simulink model "UPS_Harness"  (R2025b)
settings: Solver=VariableStepAuto  StartTime=0.0  StopTime=10.0  RelTol=1e-3
PreLoadFcn:
  | UPSHarnessParam
undefined symbols (not defined in the file): ctLimitDelayTime, DiscIntNeverNeededParam, ee_sli_rtmsupport, gcbh, powerTau, Ts, ups
libraries: eeGeneralControl x18, nesl_utility x17, simulink x17, fl_lib x15, ee_lib x13, eeTransforms x7, nesl_utility_internal x4, slpidlib x3, eeSinusoidalMeasurementV2 x3, simulink_extras x3, batteryecm_lib x1
(part 1 of 3)
settings Model: SimulationMode=accelerator  Creator=skota  LastModifiedBy=skota
settings SimscapeCC: SimscapeNominalValues="[{\"value\":\"1\",\"unit\":\"A\"},{\"value\":\"1\",\"unit\":\"bar\"},{\"value\":\"1\",\"unit\":\"cm^2\"},{\"value\":\"1\",\"unit\":\"cm^3/s\"},{\"value\":\"1\",\"unit\":\"kJ/kg\"},{\"value\":\"1\",\"unit\":\"kW\"},{\"value\":\"1\",\"unit\":\"l\"},{\"value\":\"1\",\"unit\":\"N\"},{\"value\":\"1\",\"unit\":\"N*m\"},{\"value\":\"1\",\"unit\":\"V\"},{\"value\":\"0.001\",\"unit\":\"Wb\"}]"  SimscapeLogType=all  SimscapeLogDataHistory=10000.0

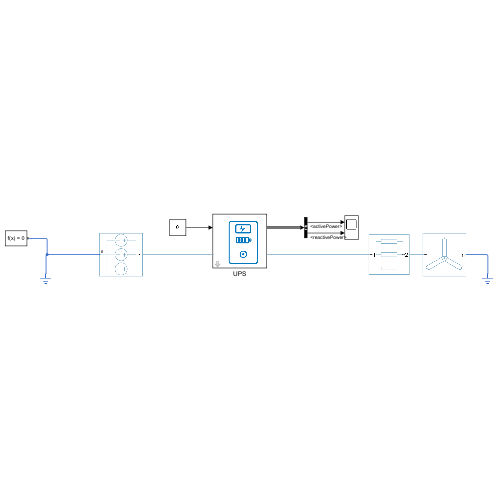
[thumbnail: Simulink's stored preview of the top-level diagram]
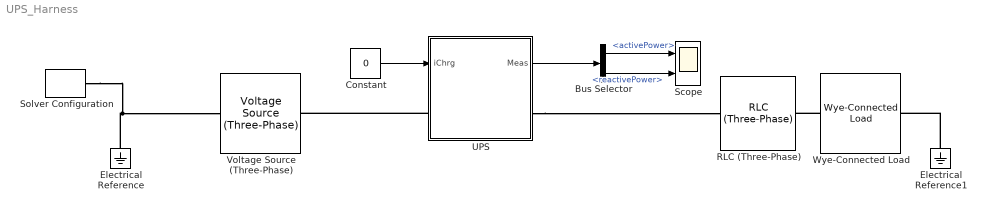
== system UPS_Harness ==
  Bus Selector : BusSelector  OutputSignals=activePower,reactivePower
  Constant : Constant  Value=0
  Electrical Reference : fl_lib/Electrical/Electrical Elements/Electrical Reference
  Electrical Reference1 : fl_lib/Electrical/Electrical Elements/Electrical Reference
  RLC (Three-Phase) : ee_lib/Passive/RLC Assemblies/RLC (Three-Phase)  port_option=ee.enum.threePhasePort.composite  component_structure=ee.enum.rlc.structure.SeriesRL  R=1e-3%1e-4 Ohm  L=1e-6%1e-6 H  C=1e-6 F  R_parasitic=0 Ohm  G_parasitic=0 1/Ohm  IL_specify=on  IL_priority=None  IL=[0, 0, 0] A  IL_nominal_specify=off  IL_nominal_value=1  IL_nominal_unit=A  VC_specify=off  VC_priority=High  VC=[0, 0, 0] V  VC_nominal_specify=off  VC_nominal_value=1  VC_nominal_unit=V
      settings: InternalSimscapePortConfiguration="{\"Bottom\":[],\"Left\":[{\"id\":\"N1\",\"label\":\"~1\",\"type\":\"foundation.electrical.three_phase\"}],\"Right\":[{\"id\":\"N2\",\"label\":\"~2\",\"type\":\"foundation.electrical.three_phase\"}],\"Top\":[]}"
  Scope : Scope  NumInputPorts=2
      settings: ActiveDisplayYMinimum=-0.21717688622608089  ActiveDisplayYMaximum=1.9545919760347286
  Solver Configuration : nesl_utility/Solver Configuration  PhysicalDomain=network_engine_domain  SubClassName=solver  LeftPortType=input  RightPortType=generic  Tones=[]  Harmonics=[]  SimulateNoise=off  Profile=off  UseLocalSampling=off  EnableSwitchedLinearOptims=on  FrequencyDomain=off  UseCCode=off  RelTol=0.001  AbsTol=0.001  MinStep=1e-09  ToWorkspace=off  RevertToSquareIcSolve=off  NumHomotopyIterations=100  PhasorMode=off  PhasorModeNumHarmonics=1  ConsistencySolver=NEWTON_XTOL_AFTER_FTOL  IndexReductionMethod=None  DoDC=off  ResidualTolerance=1e-09  ConsistencyTolSource=GLOBAL  ConsistencyAbsTol=0.001  ConsistencyRelTol=0.001  ConsistencyTolFactor=1e3  UseLocalSolver=on  LocalSolverChoice=NE_BACKWARD_EULER_ADVANCER  ResolveIndetEquations=off  FunctionEvalNumThread=1  LocalSolverSampleTime=5e-05  DoFixedCost=on  MaxNonlinIter=1  MaxModeIter=2  ComputeImpulses=off  ImpulseIterations=2  LinearAlgebra=auto  LinearAlgebraNumThread=0  EquationFormulation=NE_TIME_EF  DelaysMemoryBudget=1024  AutomaticFiltering=off  FilteringTimeConstant=0.001  PartitionStorageMethod=AS_NEEDED  PartitionMemoryBudget=1024  PartitionMethod=ROBUST  MultibodyUseLocalSolver=off  MultibodyLocalSolverChoice=ODE1  MultibodyLocalSolverSampleTime=0.001
  UPS : Subsystem  VariantControl=Detailed  mask(Double-conversion Uniterrupted Power Supply (UPS)){plantRating=ups.rating, Vac=ups.Vac, frequency=ups.frequency, baseVoltageDC=ups.Vdc, sampleTime=ups.sampleTime, filterInductanceAFE=ups.AFE.filterInductance, filterResistanceAFE=ups.AFE.filterResistance/10, capacitance=ups.DCBus.capacitance, vBattNom=ups.batt.Vnom, iBatt=ups.batt.iRated, vBattMax=ups.batt.VMax, droopGain=ups.DCBus.droop, rampRate=ups.batt.rampRate, vGridMin=ups.DCBus.gridThreshold, vDCThreshold=ups.DCBus.VThreshold, initialMode=ups.batt.initialMode, kpDC=500%ups.DCBus.kpConverter/10, kiDC=500%ups.DCBus.kiConverter/10, bessConverterEfficiency=ups.DCBus.converterEff, filterInductance=ups.inverter.filterInductance, filterResistance=ups.inverter.filterResistance}
      mask prompts: plantRating "UPS Rating (kW)"; Vac "Rated AC side voltage (phase-phase RMS) (V)"; frequency "Rated electrical frequency at AC side (Hz)"; baseVoltageDC "Voltage on DC side (V)"; sampleTime "Sample time (s)"; filterInductanceAFE "Filter inductance (H)"; filterResistanceAFE "Filter resistance (Ohm)"; capacitance "Capacitance (F)"; vBattNom "Battery nominal voltage (V)"; iBatt "Battery rated current (A)"; vBattMax "Maximum battery voltage (V)"; droopGain "DC bus droop gain"; rampRate "Ramp rate for battery discharge"; vGridMin "Minimum grid voltage (V)"; vDCThreshold "Threshold DC Bus voltage (V)"; initialMode "Initial operating mode"; kpDC "DC-DC Converter proportional gain"; kiDC "DC-DC Converter integral gain"; bessConverterEfficiency "DC-DC converter efficiency (%)"; filterInductance "Filter inductance (H)"; filterResistance "Filter series resistance (Ohm)"
      mask help: This block models a double conversion uninterruptible power supply that continuously supplies the load through an inverter. It isolates the load from input disturbances and uses a battery on the DC link to maintain uninterrupted power during input outages.
      mask Help: web('UPS.html')
      mask DialogControl generalDetailed Prompt: General
      mask DialogControl Container9 Prompt: Active Front End
      mask DialogControl editRectifier Prompt: Edit converter parameters
      mask DialogControl editRectifier Callback:
      | blockPath = [gcb,'/','Rectifier','/','AC-DC Converter'];
      |     component.mask.openBlock(blockPath);
      mask DialogControl configureAFEController Prompt: Edit AFE controller
      mask DialogControl configureAFEController Callback:
      | blockPath = [gcb,'/','Rectifier','/','PFC Rectifier Controller'];
      |     component.mask.openBlock(blockPath);
      mask DialogControl cellDetailed Prompt: DC Link
      mask DialogControl configureBattery Prompt: Edit battery parameters
      mask DialogControl configureBattery Callback:
      | blockPath = [gcb,'/','DC-Link','/','BESS','/','Battery'] ;
      |     component.mask.openBlock(blockPath);
      mask DialogControl controllerDetailed Prompt: Inverter
      mask DialogControl editInverter Prompt: Edit converter parameters
      mask DialogControl editInverter Callback:
      | blockPath = [gcb,'/','Inverter','/','DC- AC Converter'];
      |     component.mask.openBlock(blockPath);
      mask DialogControl editInverterController Prompt: Edit inverter controller
      mask DialogControl editInverterController Callback:
      | blockPath = [gcb,'/','Inverter','/','Inverter Controller'] ;
      |     component.mask.openBlock(blockPath);
  Voltage Source (Three-Phase) : ee_lib/Sources/Voltage Source (Three-Phase)  vline_rms=480 V  shift=0 deg  freq=60 Hz  impedance_option=1  SShortCircuit=100e6 A*V  XR=15  R=0.01 Ohm  L=3.97e-4 H  harmonic_option=0  harmonic_orders=[5, 7, 11, 13]  harmonic_ratios=[.1, .1, .1, .1]  G_parasitic=0 1/Ohm  I_specify=off  I_priority=None  I=[0, 0, 0] A  I_nominal_specify=off  I_nominal_value=1  I_nominal_unit=A
  Wye-Connected Load : ee_lib/Passive/RLC Assemblies/Wye-Connected Load  port_option=ee.enum.threePhasePort.composite  parameterization=ee.enum.rlc.parameterization.ratedpower  component_structure=ee.enum.rlc.structure.R  component_structure_PQ=ee.enum.rlc.structure.R  R=1 Ohm  L=1e-3 H  C=1e-6 F  VRated=480 V  FRated=60 Hz  P=5e6 W  Qpos=1e2 A*V  Qneg=-1e2 A*V  R_parasitic=0 Ohm  G_parasitic=0 1/Ohm  R_parasitic_PQ=0 Ohm  G_parasitic_PQ=0 1/Ohm  Vmag0=24e3 V  Vang0=0 deg  Freq0=60 Hz  IL_specify=off  IL_priority=High  IL=[0, 0, 0] A  IL_nominal_specify=off  IL_nominal_value=1  IL_nominal_unit=A  VC_specify=off  VC_priority=High  VC=[0, 0, 0] V  VC_nominal_specify=off  VC_nominal_value=1  VC_nominal_unit=V
  wires:
  Constant/1 -> UPS/1(iChrg)
  UPS/1(Meas) -> Bus Selector/1
  Bus Selector/1 -> Scope/1  "<activePower>"
  Bus Selector/2 -> Scope/2  "<reactivePower>"
  connections:
  UPS/LConn1 -- Voltage Source (Three-Phase)/RConn1
  Electrical Reference/LConn1 -- Solver Configuration/RConn1 -- Voltage Source (Three-Phase)/LConn1
  UPS/RConn1 -- RLC (Three-Phase)/LConn1
  Wye-Connected Load/LConn1 -- RLC (Three-Phase)/RConn1
  Electrical Reference1/LConn1 -- Wye-Connected Load/RConn1

== system UPS_Harness/UPS ==
  iChrg : Inport
  DC-Link : Subsystem
      settings: CopyFcn=set_param(gcbh,'LinkStatus','none');
      mask Display: image('DCBusbattery_1_1.png');
  Inverter : Subsystem
      settings: PortSchema="{\"entries\":[{\"content\":{\"sides\":[{\"content\":{\"connectorIds\":[\"LConn1\",\"Out1\"]},\"type\":\"ConnectorPlacement.EquallySpacedRectSide\",\"uuid\":\"30eca24e-4a0d-4322-ab8d-7623f6b77d91\"},{\"content\":{\"connectorIds\":[\"In1\",\"RConn1\",\"RConn2\"],\"side\":\"RIGHT\"},\"type\":\"ConnectorPlacement.EquallySpacedRectSide\",\"uuid\":\"08a32252-dd7d-4c32-87e9-6b7a03d2f0b7\"},{\"content\":{\"side\":\"TOP\"},\"type\":\"ConnectorPlacement.EquallySpacedRectSide\",\"uuid\":\"b32a0ebb-b906-46f8-8fa8-e8ceac70a0fa\"}]},\"type\":\"ConnectorPlacement.EquallySpacedConnector\",\"uuid\":\"2dde14a6-acee-4d4e-9286-e85271f40ce0\"}],\"packageUris\":[\"http://schema.mathworks.com/mf0/Connector/R2020b\"],\"version\":\"1.0\"}"
      mask Display: image('Copy_2_of_Inverter.png');
  Rectifier : Subsystem
      mask Display: image('rectifier_1_1.png');
  ABC : PMIOPort  Side=Left
  ~ : PMIOPort  Port=2  Side=Right
  Meas : Outport
  wires:
  DC-Link/1(Meas) -> Rectifier/1(Meas), Inverter/1(DCMeas)
  Rectifier/1(Id) -> DC-Link/2(iPFC)
  iChrg/1 -> DC-Link/1(iChrg)
  Inverter/1(Meas) -> Meas/1
  Rectifier/2(V) -> DC-Link/3(vPCC)
  Rectifier/3(Brk) -> DC-Link/4(Brk)
  connections:
  Rectifier/RConn1 -- DC-Link/LConn1
  Rectifier/RConn2 -- DC-Link/LConn2
  Rectifier/LConn1 -- ABC/RConn1
  Inverter/LConn1 -- ~/RConn1
  DC-Link/RConn1 -- Inverter/RConn1
  Inverter/RConn2 -- DC-Link/RConn2

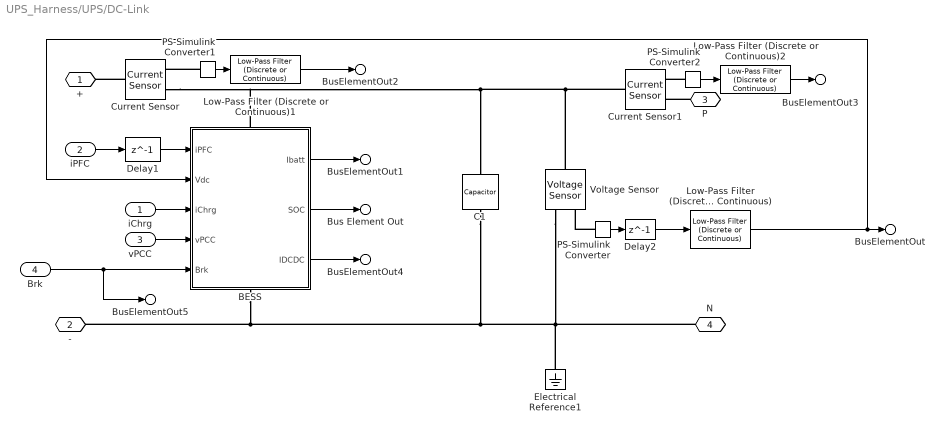
== system UPS_Harness/UPS/DC-Link ==
  iChrg : Inport
  iPFC : Inport  Port=2
  vPCC : Inport  Port=3
  Brk : Inport  Port=4
  BESS : Subsystem
      settings: PortSchema="{\"entries\":[{\"content\":{\"sides\":[{\"content\":{\"connectorIds\":[\"LConn1\"]},\"type\":\"ConnectorPlacement.EquallySpacedRectSide\",\"uuid\":\"dc16109c-3681-46df-aa2d-40033a424f4f\"},{\"content\":{\"connectorIds\":[\"RConn1\"],\"side\":\"RIGHT\"},\"type\":\"ConnectorPlacement.EquallySpacedRectSide\",\"uuid\":\"5490aea4-59f2-45ea-9bac-3971cd260353\"},{\"content\":{\"connectorIds\":[\"Out1\",\"Out2\",\"Out3\"],\"side\":\"TOP\"},\"type\":\"ConnectorPlacement.EquallySpacedRectSide\",\"uuid\":\"92b5185c-680a-4a4f-a590-9680bdd408ad\"},{\"content\":{\"connectorIds\":[\"In1\",\"In2\",\"In3\",\"In4\",\"In5\"],\"side\":\"BOTTOM\"},\"type\":\"ConnectorPlacement.EquallySpacedRectSide\",\"uuid\":\"bb2f2b82-1e61-49ed-8567-aad9343e236f\"}]},\"type\":\"ConnectorPlacement.EquallySpacedConnector\",\"uuid\":\"c23d7033-d24f-41ec-a8dd-f02fcfba4177\"}],\"packageUris\":[\"http://schema.mathworks.com/mf0/Connector/R2020b\"],\"version\":\"1.0\"}"
  C1 : fl_lib/Electrical/Electrical Elements/Capacitor  c=capacitance F  r=1e-3 Ohm  g=0 1/Ohm  i_specify=on  i_priority=None  i=0 A  i_nominal_specify=off  i_nominal_value=1  i_nominal_unit=A  v_specify=off  v_priority=High  v=0 V  v_nominal_specify=off  v_nominal_value=1  v_nominal_unit=V  vc_specify=on  vc_priority=None  vc=baseVoltageDC V  vc_nominal_specify=off  vc_nominal_value=1  vc_nominal_unit=V
  Current Sensor : fl_lib/Electrical/Electrical Sensors/Current Sensor
  Current Sensor1 : fl_lib/Electrical/Electrical Sensors/Current Sensor
  Delay1 : Delay  DelayLength=1  InitialCondition=0.5
  Delay2 : Delay  DelayLength=1  InitialCondition=baseVoltageDC
  Electrical Reference1 : fl_lib/Electrical/Electrical Elements/Electrical Reference
  Low-Pass Filter (Discrete or Continuous) : eeGeneralControl/Low-Pass Filter (Discrete or Continuous)  K=1  T=0.001  B=inf  A=-inf  init_option=Inherited from block input  x0=0  Ts=-1
  Low-Pass Filter (Discrete or Continuous)1 : eeGeneralControl/Low-Pass Filter (Discrete or Continuous)  K=1  T=0.001  B=inf  A=-inf  init_option=Inherited from block input  x0=0  Ts=-1
  Low-Pass Filter (Discrete or Continuous)2 : eeGeneralControl/Low-Pass Filter (Discrete or Continuous)  K=1  T=0.001  B=inf  A=-inf  init_option=Inherited from block input  x0=0  Ts=-1
  PS-Simulink Converter : nesl_utility/PS-Simulink Converter  PhysicalDomain=network_engine_domain  SubClassName=ps_output  LeftPortType=input  RightPortType=output  PseudoPeriodic=off  Frequencies=[]  VectorFormat=inherit  Unit=inherit  AffineConversion=off
  PS-Simulink Converter1 : nesl_utility/PS-Simulink Converter  PhysicalDomain=network_engine_domain  SubClassName=ps_output  LeftPortType=input  RightPortType=output  PseudoPeriodic=off  Frequencies=[]  VectorFormat=inherit  Unit=inherit  AffineConversion=off
  PS-Simulink Converter2 : nesl_utility/PS-Simulink Converter  PhysicalDomain=network_engine_domain  SubClassName=ps_output  LeftPortType=input  RightPortType=output  PseudoPeriodic=off  Frequencies=[]  VectorFormat=inherit  Unit=inherit  AffineConversion=off
  Voltage Sensor : fl_lib/Electrical/Electrical Sensors/Voltage Sensor
  + : PMIOPort  Side=Left
  - : PMIOPort  Port=2  Side=Left
  P : PMIOPort  Port=3  Side=Right
  N : PMIOPort  Port=4  Side=Right
  Bus Element Out : Outport  PortName=Meas  Element=SOC
  BusElementOut : Outport  PortName=Meas  Element=Vdc
  BusElementOut1 : Outport  PortName=Meas  Element=Ibatt
  BusElementOut2 : Outport  PortName=Meas  Element=Idc
  BusElementOut3 : Outport  PortName=Meas  Element=ILoad
  BusElementOut4 : Outport  PortName=Meas  Element=IDCDC
  BusElementOut5 : Outport  PortName=Meas  Element=UPSBrK
  wires:
  iPFC/1 -> Delay1/1
  Delay2/1 -> Low-Pass Filter (Discrete or Continuous)/1
  iChrg/1 -> BESS/3(iChrg)
  Delay1/1 -> BESS/1(iPFC)
  PS-Simulink Converter/1 -> Delay2/1
  BESS/1(Ibatt) -> BusElementOut1/1
  vPCC/1 -> BESS/4(vPCC)
  Brk/1 -> BusElementOut5/1, BESS/5(Brk)
  BESS/2(SOC) -> Bus Element Out/1
  Low-Pass Filter (Discrete or Continuous)/1 -> BESS/2(Vdc), BusElementOut/1
  PS-Simulink Converter1/1 -> Low-Pass Filter (Discrete or Continuous)1/1
  PS-Simulink Converter2/1 -> Low-Pass Filter (Discrete or Continuous)2/1
  Low-Pass Filter (Discrete or Continuous)2/1 -> BusElementOut3/1
  Low-Pass Filter (Discrete or Continuous)1/1 -> BusElementOut2/1
  BESS/3(IDCDC) -> BusElementOut4/1
  connections:
  Electrical Reference1/LConn1 -- N/RConn1 -- Voltage Sensor/RConn2 -- C1/RConn1 -- BESS/RConn1 -- -/RConn1
  PS-Simulink Converter/LConn1 -- Voltage Sensor/RConn1
  Voltage Sensor/LConn1 -- Current Sensor1/LConn1 -- C1/LConn1 -- Current Sensor/RConn2 -- BESS/LConn1
  PS-Simulink Converter1/LConn1 -- Current Sensor/RConn1
  P/RConn1 -- Current Sensor1/RConn2
  PS-Simulink Converter2/LConn1 -- Current Sensor1/RConn1
  Current Sensor/LConn1 -- +/RConn1

== system UPS_Harness/UPS/Inverter ==
  DCMeas : Inport
  DC- AC Converter : ee_lib/Semiconductors & Converters/Converters/Average-Value Voltage Source Converter (Three-Phase)  port_option=ee.enum.threePhasePort.composite  frequency_option=ee.enum.converters.frequency.variable  input_option=ee.enum.converters.inputOption.ModWave  FRated=60 Hz  losses_parameterization=ee.enum.converters.losses.fixed  Pfixed=0.5 W  ks=0.01  kc1=1.7 V  kc2=0.01 Ohm  Ploss_vect=[100, 800, 1870, 3250, 4900] W  Irms_vect=[10, 100, 200, 300, 400] A  Vdc_nom=300 V  thermal_mass=30000 J/K  temperature_specify=off  temperature_priority=High  temperature=298.15 K  temperature_nominal_specify=off  temperature_nominal_value=1  temperature_nominal_unit=K
      settings: InternalSimscapePortConfiguration="{\"Bottom\":[],\"Left\":[{\"id\":\"ModWave\",\"label\":\"ModWave\",\"type\":\"input\"},{\"id\":\"N\",\"label\":\"~\",\"type\":\"foundation.electrical.three_phase\"}],\"Right\":[{\"id\":\"p\",\"label\":\"+\",\"type\":\"foundation.electrical.electrical\"},{\"id\":\"n\",\"label\":\"-\",\"type\":\"foundation.electrical.electrical\"}],\"Top\":[]}"
  Filter & Measurements : Subsystem
      settings: PortSchema="{\"entries\":[{\"content\":{\"sides\":[{\"content\":{\"connectorIds\":[\"LConn1\",\"In1\"]},\"type\":\"ConnectorPlacement.EquallySpacedRectSide\",\"uuid\":\"460c57c7-bd36-455c-a026-acc96216539a\"},{\"content\":{\"connectorIds\":[\"Out1\",\"Out2\",\"RConn1\"],\"side\":\"RIGHT\"},\"type\":\"ConnectorPlacement.EquallySpacedRectSide\",\"uuid\":\"ae96aff3-eaea-4e67-97f2-c12a1605f490\"},{\"content\":{\"side\":\"TOP\"},\"type\":\"ConnectorPlacement.EquallySpacedRectSide\",\"uuid\":\"723b0a2f-7df5-41f2-b267-8daf9f0832d8\"}]},\"type\":\"ConnectorPlacement.EquallySpacedConnector\",\"uuid\":\"b3aac9a5-3f98-4392-99ca-65ef3ff3ee74\"}],\"packageUris\":[\"http://schema.mathworks.com/mf0/Connector/R2020b\"],\"version\":\"1.0\"}"
  Inverter Controller : Subsystem  VariantControl=Grid Forming  mask(UPS Controller){measSampleTime=ups.sampleTime, dcBusVoltage=baseVoltageDC, powerFreq=frequency, girdLineVoltage=Vac, power=plantRating*1000, fDroop=ups.inverter.fDroop, vDroop=ups.inverter.vDroop, vdPGain=ups.inverter.kpVd, VdIGain=ups.inverter.kiVd, VdMaxCt=ups.inverter.IMaxVd, VqPGain=ups.inverter.kpVq, VqIGain=ups.inverter.kiVq, VqMaxCt=ups.inverter.IMaxVd, VdMinCt=ups.inverter.IMinVd, VqMinCt=ups.inverter.IMinVd, vdvqLPFTimeConst=ups.sampleTime*100, voltControlTs=ups.sampleTime, currentControlTs=ups.sampleTime, IdPGain=ups.inverter.kpId, IdIGain=ups.inverter.kiId, IqPGain=ups.inverter.kpIq, IqIGain=ups.inverter.kiIq, filterInductance=filterInductance, currentLimitMethod=Virtual impedance, maxSatCurrentLimit=ups.iLimit.value, ctLimitXbyR=ups.iLimit.XByR, ctLimitVirtualImp=ups.iLimit.resistance}
      mask prompts: measSampleTime "Measurement sample time"; dcBusVoltage "DC bus voltage"; powerFreq "Grid frequency (Hz)"; girdLineVoltage "Grid line voltage (V)"; power "Converter power (VA)"; fDroop "Frequency droop"; vDroop "Voltage droop"; vdPGain "Vd proportional gain"; VdIGain "Vd integral gain"; VdMaxCt "Vd maximum current limit (A)"; VqPGain "Vq proportional gain"; VqIGain "Vq integral gain"; VqMaxCt "Vq maximum current limit (A)"; VdMinCt "Vd minimum current limit  (A)"; VqMinCt "Vq minimum current limit  (A)"; vdvqLPFTimeConst "Voltage measurement filter time constant (s)"; voltControlTs "Controller sample time (s)"; currentControlTs "Controller sample time (s)"; IdPGain "Id proportional gain"; IdIGain "Id integral gain"; IqPGain "Iq proportional gain"; IqIGain "Iq integral gain"; filterInductance "Filter inductance (H)"; currentLimitMethod "Current limiting method"; maxSatCurrentLimit "Maximum current limit (pu)"; ctLimitXbyR "Virtual X/R ratio"; ctLimitVirtualImp "Virtual impedance co-efficient (pu.Ohm/pu.A)"
      mask help: This block implements the uniterrupted power supply inverter control
      settings: CopyFcn=set_param(gcb,'LinkStatus','none');
      mask TypeOptions currentLimitMethod: Virtual impedance | Current saturation
      mask Callback currentLimitMethod: component.mask.iLimitSelection;
      mask DialogControl Container7 Prompt: General
      mask DialogControl Container9 Prompt: Voltage Control
      mask DialogControl Container10 Prompt: Current Control
      mask DialogControl Container8 Prompt: Current Limiting
  Simulink-PS Converter : nesl_utility/Simulink-PS Converter  PhysicalDomain=network_engine_domain  SubClassName=ps_input  LeftPortType=input  RightPortType=output  PseudoPeriodic=off  Frequencies=[]  NoiseDistribution=none  NoiseParameters=[]  Unit=1  AffineConversion=off  FilteringAndDerivatives=provide  SimscapeFilterOrder=1  InputFilterTimeConstant=0.001  UdotUserProvided=0
  ~ : PMIOPort  Side=Left
  + : PMIOPort  Port=2  Side=Right
  - : PMIOPort  Port=3  Side=Right
  Meas : Outport
  wires:
  Inverter Controller/1(mabc) -> Simulink-PS Converter/1
  DCMeas/1 -> Filter & Measurements/1(DCBusMeas)
  Filter & Measurements/1(VIBus) -> Inverter Controller/1(VI)
  Filter & Measurements/2(Meas) -> Inverter Controller/2(Power), Meas/1
  connections:
  DC- AC Converter/RConn2 -- -/RConn1
  +/RConn1 -- DC- AC Converter/RConn1
  Simulink-PS Converter/RConn1 -- DC- AC Converter/LConn1
  DC- AC Converter/LConn2 -- Filter & Measurements/LConn1
  ~/RConn1 -- Filter & Measurements/RConn1

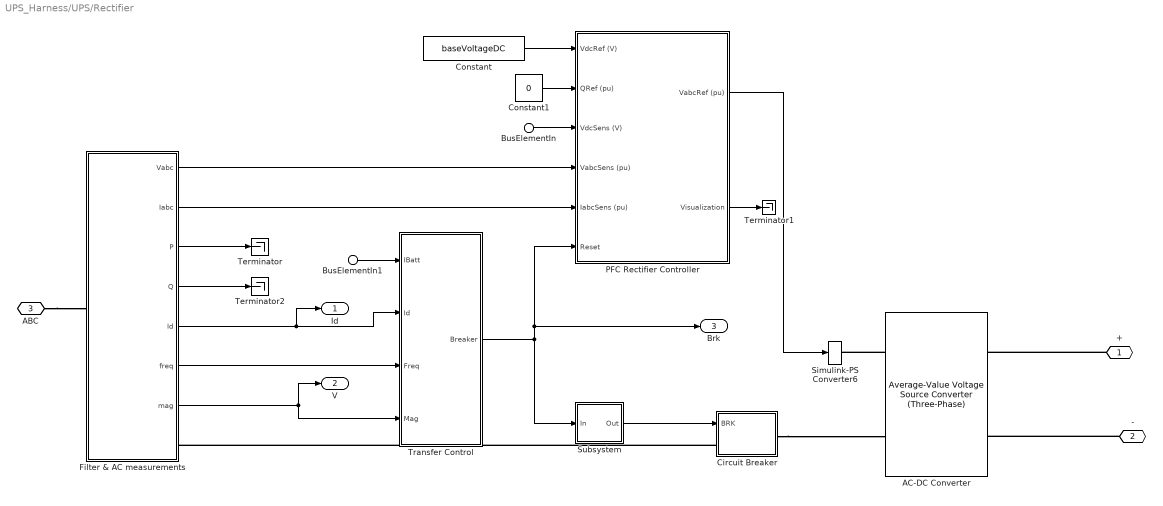
== system UPS_Harness/UPS/Rectifier ==
  BusElementIn : Inport  PortName=Meas  Element=Vdc
  BusElementIn1 : Inport  PortName=Meas  Element=Ibatt
  AC-DC Converter : ee_lib/Semiconductors & Converters/Converters/Average-Value Voltage Source Converter (Three-Phase)  port_option=ee.enum.threePhasePort.composite  frequency_option=ee.enum.converters.frequency.variable  input_option=ee.enum.converters.inputOption.ModWave  FRated=60 Hz  losses_parameterization=ee.enum.converters.losses.fixed  Pfixed=1 W  ks=0.01  kc1=1.7 V  kc2=0.01 Ohm  Ploss_vect=[100, 800, 1870, 3250, 4900] W  Irms_vect=[10, 100, 200, 300, 400] A  Vdc_nom=300 V  thermal_mass=30000 J/K  temperature_specify=off  temperature_priority=High  temperature=298.15 K  temperature_nominal_specify=off  temperature_nominal_value=1  temperature_nominal_unit=K
      settings: InternalSimscapePortConfiguration="{\"Bottom\":[],\"Left\":[{\"id\":\"ModWave\",\"label\":\"ModWave\",\"type\":\"input\"},{\"id\":\"N\",\"label\":\"~\",\"type\":\"foundation.electrical.three_phase\"}],\"Right\":[{\"id\":\"p\",\"label\":\"+\",\"type\":\"foundation.electrical.electrical\"},{\"id\":\"n\",\"label\":\"-\",\"type\":\"foundation.electrical.electrical\"}],\"Top\":[]}"
  Circuit Breaker : Subsystem
  Constant : Constant  Value=baseVoltageDC
  Constant1 : Constant  Value=0
  Filter & AC measurements : Subsystem
  PFC Rectifier Controller : Subsystem  LoadFcn=%ee_sli_rtmsupport( 'loadfcn', gcbh );  mask(PFC Rectifier Controller (Three-Phase)){Freq=frequency, L=ups.AFE.filterInductance, BaseImpedance=Vac*Vac/(plantRating*1000), KpPLL=ups.AFE.kpPLL, KiPLL=ups.AFE.kiPLL, Ts=-1, KpVoltage=ups.AFE.kpVoltage, KiVoltage=ups.AFE.kiVoltage, KdVoltage=ups.AFE.kdVoltage, NdVoltage=ups.AFE.derivativeFilter, BaseVdc=baseVoltageDC, VoltControlUpperLimit=ups.AFE.voltageUpperLimit, VoltControlLowerLimit=ups.AFE.voltageLowerLimit, KpdCurrent=ups.AFE.kpId/50, KidCurrent=ups.AFE.kiId, KddCurrent=ups.AFE.kdId, IdControlUpperLimit=ups.AFE.IdUpperLimit, IdControlLowerLimit=ups.AFE.IdLowerLimit, KpqCurrent=ups.AFE.kpIq/50, KiqCurrent=ups.AFE.kiIq, KdqCurrent=ups.AFE.kdIq, NdCurrent=ups.AFE.derivativeFilter, IqControlUpperLimit=ups.AFE.IqUpperLimit, IqControlLowerLimit=ups.AFE.IqLowerLimit}
      mask prompts: Freq "physmod:ee:library:comments:control:eeConverterControllers:SystemFrequencyHz_MP"; L "physmod:ee:library:comments:control:eeConverterControllers:ACFilterInductanceH_MP"; BaseImpedance "physmod:ee:library:comments:control:eeConverterControllers:ACSideBaseImpedanceOhm_MP"; KpPLL "physmod:ee:library:comments:control:eeConverterControllers:PLLProportionalGain_MP"; KiPLL "physmod:ee:library:comments:control:eeConverterControllers:PLLIntegralGain_MP"; Ts "physmod:ee:library:comments:control:eeConverterControllers:SampleTime1ForInherited_MP"; KpVoltage "physmod:ee:library:comments:control:eeConverterControllers:ProportionalGain_MP"; KiVoltage "physmod:ee:library:comments:control:eeConverterControllers:IntegralGain_MP"; KdVoltage "physmod:ee:library:comments:control:eeConverterControllers:DerivativeGain_MP"; NdVoltage "physmod:ee:library:comments:control:eeConverterControllers:DerivativeControllerFilterCoefficientN_MP"; BaseVdc "physmod:ee:library:comments:control:eeConverterControllers:DCBusBaseVoltageV_MP"; VoltControlUpperLimit "physmod:ee:library:comments:control:eeConverterControllers:ControllerOutputUpperLimitpu_MP"; VoltControlLowerLimit "physmod:ee:library:comments:control:eeConverterControllers:ControllerOutputLowerLimitpu_MP"; KpdCurrent "physmod:ee:library:comments:control:eeConverterControllers:IdProportionalGain_MP"; KidCurrent "physmod:ee:library:comments:control:eeConverterControllers:IdIntegralGain_MP"; KddCurrent "physmod:ee:library:comments:control:eeConverterControllers:IdDerivativeGain_MP"; IdControlUpperLimit "physmod:ee:library:comments:control:eeConverterControllers:IdControllerOutputUpperLimitpu_MP"; IdControlLowerLimit "physmod:ee:library:comments:control:eeConverterControllers:IdControllerOutputLowerLimitpu_MP"; KpqCurrent "physmod:ee:library:comments:control:eeConverterControllers:IqProportionalGain_MP"; KiqCurrent "physmod:ee:library:comments:control:eeConverterControllers:IqIntegralGain_MP"; KdqCurrent "physmod:ee:library:comments:control:eeConverterControllers:IqDerivativeGain_MP"; NdCurrent "physmod:ee:library:comments:control:eeConverterControllers:DerivativeCurrentControllerFilterCoefficientN_MP"; IqControlUpperLimit "physmod:ee:library:comments:control:eeConverterControllers:IqControllerOutputUpperLimitpu_MP"; IqControlLowerLimit "physmod:ee:library:comments:control:eeConverterControllers:IqControllerOutputLowerLimitpu_MP"
      mask help: physmod:ee:library:comments:control:eeConverterControllers:PFCRectifierController_MD
      mask init:
      | ee.mask.initializePFCController(gcb,Ts, Freq, L,BaseImpedance,KpPLL,KiPLL,KpVoltage,KiVoltage,KdVoltage,BaseVdc, NdVoltage,VoltControlUpperLimit,VoltControlLowerLimit,KpdCurrent, KidCurrent, KddCurrent, NdCurrent, IdControlUpperLimit, IdControlLowerLimit, KpqCurrent, KiqCurrent, KdqCurrent, IqControlUpperLimit, IqControlLowerLimit);
      settings: CopyFcn=%ee_sli_rtmsupport( 'copyfcn', gcbh );  DeleteFcn=ee_sli_rtmsupport( 'deletefcn', gcbh );  ModelCloseFcn=ee_sli_rtmsupport( 'modelclosefcn', gcbh );  PostSaveFcn=ee_sli_rtmsupport( 'postsavefcn', gcbh );  PreCopyFcn=ee_sli_rtmsupport( 'precopyfcn', gcbh );  OpenFcn=ee_sli_rtmsupport( 'openfcn', gcbh );  CloseFcn=%ee_sli_rtmsupport( 'closefcn', gcbh );  PreDeleteFcn=ee_sli_rtmsupport( 'predeletefcn', gcbh );
      mask Help: web(nesl_help(gcbh))
      mask DialogControl GeneralTabVal Prompt: physmod:ee:library:comments:control:eeConverterControllers:tab_General
      mask DialogControl Freq Prompt: System frequency (Hz)
      mask DialogControl L Prompt: AC filter inductance (H)
      mask DialogControl BaseImpedance Prompt: AC side base impedance (Ohm)
      mask DialogControl KpPLL Prompt: PLL proportional gain
      mask DialogControl KiPLL Prompt: PLL integral gain
      mask DialogControl Ts Prompt: Sample time (-1 for inherited)
      mask DialogControl VoltageControl Prompt: physmod:ee:library:comments:control:eeConverterControllers:tab_VoltageController
      mask DialogControl KpVoltage Prompt: Proportional gain
      mask DialogControl KiVoltage Prompt: Integral gain
      mask DialogControl KdVoltage Prompt: Derivative gain
      mask DialogControl NdVoltage Prompt: Derivative controller filter coefficient (N)
      mask DialogControl BaseVdc Prompt: DC bus base voltage (V)
      mask DialogControl VoltControlUpperLimit Prompt: Controller output upper limit (pu)
      mask DialogControl VoltControlLowerLimit Prompt: Controller output lower limit (pu)
      mask DialogControl CurrentControl Prompt: physmod:ee:library:comments:control:eeConverterControllers:tab_CurrentController
      mask DialogControl KpdCurrent Prompt: Id proportional gain
      mask DialogControl KidCurrent Prompt: Id integral gain
      mask DialogControl KddCurrent Prompt: Id derivative gain
      mask DialogControl IdControlUpperLimit Prompt: Id controller output upper limit (pu)
      mask DialogControl IdControlLowerLimit Prompt: Id controller output lower limit (pu)
      mask DialogControl KpqCurrent Prompt: Iq proportional gain
      mask DialogControl KiqCurrent Prompt: Iq integral gain
      mask DialogControl KdqCurrent Prompt: Iq derivative gain
      mask DialogControl NdCurrent Prompt: Derivative current controller filter coefficient (N)
      mask DialogControl IqControlUpperLimit Prompt: Iq controller output upper limit (pu)
      mask DialogControl IqControlLowerLimit Prompt: Iq controller output lower limit (pu)
  Simulink-PS Converter6 : nesl_utility/Simulink-PS Converter  PhysicalDomain=network_engine_domain  SubClassName=ps_input  LeftPortType=input  RightPortType=output  PseudoPeriodic=off  Frequencies=[]  NoiseDistribution=none  NoiseParameters=[]  Unit=1  AffineConversion=off  FilteringAndDerivatives=provide  SimscapeFilterOrder=1  InputFilterTimeConstant=0.001  UdotUserProvided=0
  Subsystem : Subsystem
  Terminator : Terminator
  Terminator1 : Terminator
  Terminator2 : Terminator
  Transfer Control : Subsystem
  + : PMIOPort  Side=Right
  - : PMIOPort  Port=2  Side=Right
  ABC : PMIOPort  Port=3  Side=Left
  Id : Outport
  V : Outport  Port=2
  Brk : Outport  Port=3
  wires:
  Constant/1 -> PFC Rectifier Controller/1(VdcRef (V))
  Filter & AC measurements/2(Iabc) -> PFC Rectifier Controller/5(IabcSens (pu))
  Constant1/1 -> PFC Rectifier Controller/2(QRef (pu))
  PFC Rectifier Controller/2(Visualization) -> Terminator1/1
  Filter & AC measurements/1(Vabc) -> PFC Rectifier Controller/4(VabcSens (pu))
  Filter & AC measurements/3(P) -> Terminator/1
  Filter & AC measurements/4(Q) -> Terminator2/1
  Filter & AC measurements/5(Id) -> Id/1, Transfer Control/2(Id)
  BusElementIn/1 -> PFC Rectifier Controller/3(VdcSens (V))
  Filter & AC measurements/6(freq) -> Transfer Control/3(Freq)
  Filter & AC measurements/7(mag) -> V/1, Transfer Control/4(Mag)
  BusElementIn1/1 -> Transfer Control/1(IBatt)
  PFC Rectifier Controller/1(VabcRef (pu)) -> Simulink-PS Converter6/1
  Subsystem/1(Out) -> Circuit Breaker/1(BRK)
  Transfer Control/1(Breaker) -> Brk/1, PFC Rectifier Controller/6(Reset), Subsystem/1(In)
  connections:
  ABC/RConn1 -- Filter & AC measurements/LConn1
  Circuit Breaker/RConn1 -- AC-DC Converter/LConn2
  AC-DC Converter/LConn1 -- Simulink-PS Converter6/RConn1
  +/RConn1 -- AC-DC Converter/RConn1
  Circuit Breaker/LConn1 -- Filter & AC measurements/RConn1
  -/RConn1 -- AC-DC Converter/RConn2

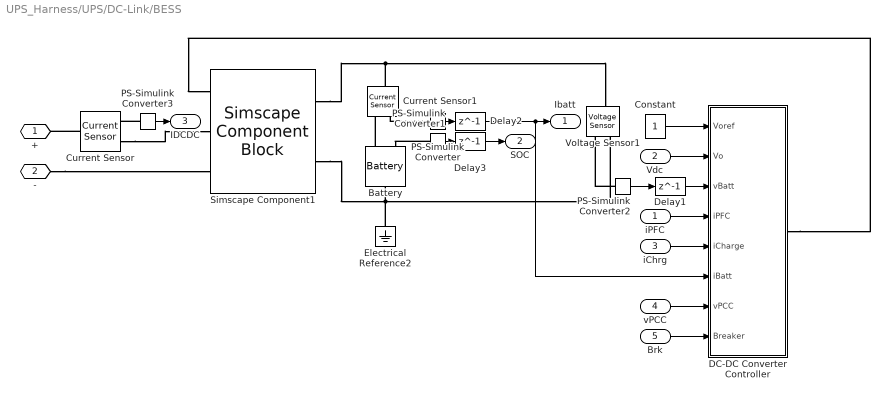
== system UPS_Harness/UPS/DC-Link/BESS ==
  iPFC : Inport
  Vdc : Inport  Port=2
  iChrg : Inport  Port=3
  vPCC : Inport  Port=4
  Brk : Inport  Port=5
  Battery : batteryecm_lib/Battery  Vnom=400 V  prm_dir=simscape.enum.battery.prm_dir.disabled  R1_dis=5e-2 Ohm  R1_ch=1e-3 Ohm  R1=1e-3 Ohm  prm_AH=simscape.enum.battery.prm_AH.infinite  AH=50 A*hr  V1=11.5 V  AH1=25 A*hr  prm_R2=simscape.enum.battery.prm_R2.disabled  R2=2000 Ohm  Tmeas=298.15 K  charge_measurement_port=simscape.enum.battery.enable.yes  prm_dyn=simscape.enum.battery.prm_dyn.off  Rp1=0.005 Ohm  tau1=30 s  Rp2=0.005 Ohm  tau2=30 s  Rp3=0.005 Ohm  tau3=30 s  Rp4=0.005 Ohm  tau4=30 s  Rp5=0.005 Ohm  tau5=30 s  prm_fade=simscape.enum.battery.prm_fade.disabled  N_fade=100  AH_fade=45 A*hr  R1_fade=2.02 Ohm  R1_ch_fade=2.02 Ohm  V1_fade=10.35 V  prm_age=simscape.enum.battery.prm_age.disabled  prm_age_OCV=simscape.enum.battery.prm_age_OCV.OCV  OCV_age=0.9  SOC_age=60  Tmeas_age=298.15 K  delta_time_age_vec=[0] d  temperature_age_vec=[273] K  OCV_scaling_age=2.2134e6  OCV_offset_age=1.632e6  temp_exp_age=0.515833569 V  t_exp_age=0.75  Vnom_T2=12 V  R1_T2=2.2 Ohm  R1_T2_dis=2.2 Ohm  R1_T2_ch=2.2 Ohm  V1_T2=11.4 V  R2_T2=2200 Ohm  Rp1_T2=0.005 Ohm  tau1_T2=30 s  Rp2_T2=0.005 Ohm  tau2_T2=30 s  Rp3_T2=0.005 Ohm  tau3_T2=30 s  Rp4_T2=0.005 Ohm  tau4_T2=30 s  Rp5_T2=0.005 Ohm  tau5_T2=30 s  Tmeas2=273.15 K  thermal_port=simscape.enum.thermaleffects.omit  thermal_mass=30000 J/K  i_specify=on  i_priority=High  i=0 A  i_nominal_specify=off  i_nominal_value=1  i_nominal_unit=A  v_specify=on  v_priority=None  v=400 V  v_nominal_specify=off  v_nominal_value=1  v_nominal_unit=V  charge_specify=on  charge_priority=None  charge=50 A*hr  charge_nominal_specify=off  charge_nominal_value=1  charge_nominal_unit=A*hr  num_cycles_specify=off  num_cycles_priority=High  num_cycles=0  num_cycles_nominal_specify=off  num_cycles_nominal_value=1  num_cycles_nominal_unit=1  temperature_specify=off  temperature_priority=High  temperature=298.15 K  temperature_nominal_specify=off  temperature_nominal_value=1  temperature_nominal_unit=K
      settings: InternalSimscapePortConfiguration="{\"Bottom\":[],\"Left\":[{\"id\":\"p\",\"label\":\"+\",\"type\":\"foundation.electrical.electrical\"},{\"id\":\"q\",\"label\":\"q\",\"type\":\"output\"}],\"Right\":[{\"id\":\"n\",\"label\":\"-\",\"type\":\"foundation.electrical.electrical\"}],\"Top\":[]}"
  Constant : Constant
  Current Sensor : fl_lib/Electrical/Electrical Sensors/Current Sensor
  Current Sensor1 : fl_lib/Electrical/Electrical Sensors/Current Sensor
  DC-DC Converter Controller : Subsystem
  Delay1 : Delay  DelayLength=1  InitialCondition=400
  Delay2 : Delay  DelayLength=1  InitialCondition=400
  Delay3 : Delay  DelayLength=1  InitialCondition=400
  Electrical Reference2 : fl_lib/Electrical/Electrical Elements/Electrical Reference
  PS-Simulink Converter{,1..3} (4 alike) : nesl_utility/PS-Simulink Converter  PhysicalDomain=network_engine_domain  SubClassName=ps_output  LeftPortType=input  RightPortType=output  PseudoPeriodic=off  Frequencies=[]  VectorFormat=inherit  Unit=inherit  AffineConversion=off
  Simscape Component1 : SimscapeComponentBlock  SourceFile=microgridRenewables.biDirectionalConverter  ComponentPath=microgridRenewables.biDirectionalConverter  ComponentVariants="[\"microgridRenewables.biDirectionalConverter\"]"  ComponentVariantNames="[\"biDirectionalConverter\"]"  ClassName=biDirectionalConverter  SchemaVersion=1  efficiency_option=ee.enum.converters.efficiency.constant  efficiency_fixed=100  i_vec=[0, 2, 5] A  efficiency_vec=[90, 95, 98]  iL_specify=off  iL_priority=High  iL=0 A  iL_nominal_specify=off  iL_nominal_value=1  iL_nominal_unit=A  vc_specify=off  vc_priority=High  vc=0 V  vc_nominal_specify=off  vc_nominal_value=1  vc_nominal_unit=V  i1_specify=off  i1_priority=None  i1=0 A  i1_nominal_specify=off  i1_nominal_value=1  i1_nominal_unit=A  i2_specify=off  i2_priority=None  i2=0 A  i2_nominal_specify=off  i2_nominal_value=1  i2_nominal_unit=A  v1_specify=off  v1_priority=None  v1=0 V  v1_nominal_specify=off  v1_nominal_value=1  v1_nominal_unit=V  v2_specify=off  v2_priority=None  v2=0 V  v2_nominal_specify=off  v2_nominal_value=1  v2_nominal_unit=V
      settings: CopyFcn=simscape.sscblock.internal.componentBlockCallback(gcbh,'COPY')  PreCopyFcn=simscape.sscblock.internal.componentBlockCallback(gcbh,'PRECOPY')  PreDeleteFcn=simscape.sscblock.internal.componentBlockCallback(gcbh,'PREDELETE')  InternalSimscapePortConfiguration="{\"Bottom\":[],\"Left\":[{\"id\":\"Iref\",\"label\":\"Iref\",\"type\":\"input\"},{\"id\":\"p1\",\"label\":\"1+\",\"type\":\"foundation.electrical.electrical\"},{\"id\":\"n1\",\"label\":\"1-\",\"type\":\"foundation.electrical.electrical\"}],\"Right\":[{\"id\":\"p2\",\"label\":\"2+\",\"type\":\"foundation.electrical.electrical\"},{\"id\":\"n2\",\"label\":\"2-\",\"type\":\"foundation.electrical.electrical\"}],\"Top\":[]}"
      mask Type: Bi-directional DC-DC Converter
  Voltage Sensor1 : fl_lib/Electrical/Electrical Sensors/Voltage Sensor
  + : PMIOPort  Side=Left
  - : PMIOPort  Port=2  Side=Right
  Ibatt : Outport
  SOC : Outport  Port=2
  IDCDC : Outport  Port=3
  wires:
  iChrg/1 -> DC-DC Converter Controller/5(iCharge)
  Vdc/1 -> DC-DC Converter Controller/2(Vo)
  Delay1/1 -> DC-DC Converter Controller/3(vBatt)
  iPFC/1 -> DC-DC Converter Controller/4(iPFC)
  Constant/1 -> DC-DC Converter Controller/1(Voref)
  PS-Simulink Converter/1 -> Delay2/1
  Delay2/1 -> Ibatt/1, DC-DC Converter Controller/6(iBatt)
  vPCC/1 -> DC-DC Converter Controller/7(vPCC)
  Brk/1 -> DC-DC Converter Controller/8(Breaker)
  PS-Simulink Converter1/1 -> Delay3/1
  Delay3/1 -> SOC/1
  PS-Simulink Converter2/1 -> Delay1/1
  PS-Simulink Converter3/1 -> IDCDC/1
  connections:
  Electrical Reference2/LConn1 -- Simscape Component1/RConn2 -- Voltage Sensor1/RConn2 -- Battery/RConn1
  Battery/LConn1 -- Current Sensor1/RConn2
  PS-Simulink Converter2/LConn1 -- Voltage Sensor1/RConn1
  -/RConn1 -- Simscape Component1/LConn3
  Current Sensor1/LConn1 -- Simscape Component1/RConn1 -- Voltage Sensor1/LConn1
  DC-DC Converter Controller/RConn1 -- Simscape Component1/LConn1
  PS-Simulink Converter/LConn1 -- Current Sensor1/RConn1
  PS-Simulink Converter1/LConn1 -- Battery/LConn2
  Current Sensor/RConn2 -- Simscape Component1/LConn2
  Current Sensor/LConn1 -- +/RConn1
  PS-Simulink Converter3/LConn1 -- Current Sensor/RConn1

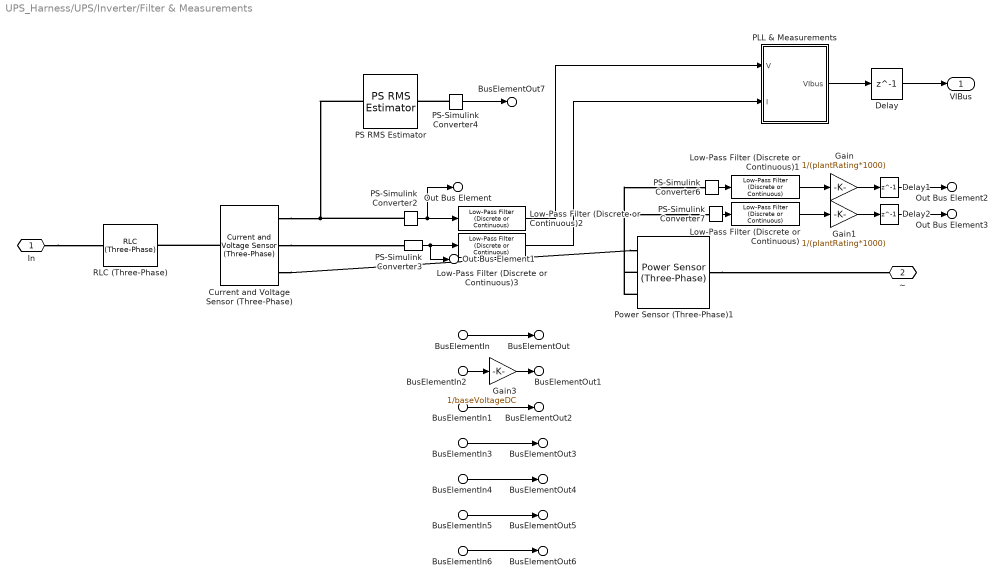
== system UPS_Harness/UPS/Inverter/Filter & Measurements ==
  BusElementIn : Inport  PortName=DCBusMeas  Element=SOC
  BusElementIn2 : Inport  PortName=DCBusMeas  Element=Vdc
  BusElementIn1 : Inport  PortName=DCBusMeas  Element=Ibatt
  BusElementIn3 : Inport  PortName=DCBusMeas  Element=Idc
  BusElementIn4 : Inport  PortName=DCBusMeas  Element=ILoad
  BusElementIn5 : Inport  PortName=DCBusMeas  Element=IDCDC
  BusElementIn6 : Inport  PortName=DCBusMeas  Element=UPSBrK
  Current and Voltage Sensor (Three-Phase) : ee_lib/Sensors & Transducers/Current and Voltage Sensor (Three-Phase)  vMeasurementType=ee.enum.vmeasurement.lg  outputUnit=ee.enum.unit.pu  SRated=plantRating*1000 A*V  VRated=Vac V  I_specify=off  I_priority=None  I=[0, 0, 0] A  I_nominal_specify=off  I_nominal_value=1  I_nominal_unit=A  V_specify=off  V_priority=None  V=[0, 0, 0] V  V_nominal_specify=off  V_nominal_value=1  V_nominal_unit=V
      settings: InternalSimscapePortConfiguration="{\"Bottom\":[],\"Left\":[{\"id\":\"N1\",\"label\":\"~1\",\"type\":\"foundation.electrical.three_phase\"}],\"Right\":[{\"id\":\"V_output\",\"label\":\"V\",\"type\":\"output\"},{\"id\":\"I_output\",\"label\":\"I\",\"type\":\"output\"},{\"id\":\"N2\",\"label\":\"~2\",\"type\":\"foundation.electrical.three_phase\"}],\"Top\":[]}"
  Delay : Delay  DelayLength=1
  Delay1 : Delay  DelayLength=1
  Delay2 : Delay  DelayLength=1
  Gain : Gain  Gain=1/(plantRating*1000)
  Gain1 : Gain  Gain=1/(plantRating*1000)
  Gain3 : Gain  Gain=1/baseVoltageDC
  Low-Pass Filter (Discrete or Continuous) : eeGeneralControl/Low-Pass Filter (Discrete or Continuous)  K=1  T=powerTau  B=inf  A=-inf  init_option=Inherited from block input  x0=0  Ts=Ts
  Low-Pass Filter (Discrete or Continuous)1 : eeGeneralControl/Low-Pass Filter (Discrete or Continuous)  K=1  T=powerTau  B=inf  A=-inf  init_option=Inherited from block input  x0=0  Ts=Ts
  Low-Pass Filter (Discrete or Continuous)2 : eeGeneralControl/Low-Pass Filter (Discrete or Continuous)  K=1  T=powerTau/10  B=inf  A=-inf  init_option=Inherited from block input  x0=0  Ts=Ts
  Low-Pass Filter (Discrete or Continuous)3 : eeGeneralControl/Low-Pass Filter (Discrete or Continuous)  K=1  T=powerTau/10  B=inf  A=-inf  init_option=Inherited from block input  x0=0  Ts=Ts
  PLL & Measurements : Subsystem
      mask Display: image('PLL_9_7_2_20_1.png');
  PS RMS Estimator : fl_lib/Physical Signals/Periodic Operators/PS RMS Estimator  f0=60 Hz
      settings: InternalSimscapePortConfiguration="{\"Bottom\":[],\"Left\":[{\"id\":\"I\",\"label\":\"\",\"type\":\"input\"}],\"Right\":[{\"id\":\"O\",\"label\":\"\",\"type\":\"output\"}],\"Top\":[]}"
  PS-Simulink Converter2 : nesl_utility_internal/PS-Simulink Converter  PhysicalDomain=network_engine_domain  SubClassName=ps_output  LeftPortType=input  RightPortType=output  PseudoPeriodic=off  Frequencies=[]  VectorFormat=1-D array  Unit=V  AffineConversion=off
  PS-Simulink Converter3 : nesl_utility_internal/PS-Simulink Converter  PhysicalDomain=network_engine_domain  SubClassName=ps_output  LeftPortType=input  RightPortType=output  PseudoPeriodic=off  Frequencies=[]  VectorFormat=1-D array  Unit=A  AffineConversion=off
  PS-Simulink Converter4 : nesl_utility/PS-Simulink Converter  PhysicalDomain=network_engine_domain  SubClassName=ps_output  LeftPortType=input  RightPortType=output  PseudoPeriodic=off  Frequencies=[]  VectorFormat=inherit  Unit=inherit  AffineConversion=off
  PS-Simulink Converter6 : nesl_utility_internal/PS-Simulink Converter  PhysicalDomain=network_engine_domain  SubClassName=ps_output  LeftPortType=input  RightPortType=output  PseudoPeriodic=off  Frequencies=[]  VectorFormat=1-D array  Unit=W  AffineConversion=off
  PS-Simulink Converter7 : nesl_utility_internal/PS-Simulink Converter  PhysicalDomain=network_engine_domain  SubClassName=ps_output  LeftPortType=input  RightPortType=output  PseudoPeriodic=off  Frequencies=[]  VectorFormat=1-D array  Unit=V*A  AffineConversion=off
  Power Sensor (Three-Phase)1 : ee_lib/Sensors & Transducers/Power Sensor (Three-Phase)  load_type=ee.enum.passive.type_balanced.balanced  f0=60 Hz
      settings: InternalSimscapePortConfiguration="{\"Bottom\":[],\"Left\":[{\"id\":\"N1\",\"label\":\"~1\",\"type\":\"foundation.electrical.three_phase\"}],\"Right\":[{\"id\":\"N2\",\"label\":\"~2\",\"type\":\"foundation.electrical.three_phase\"}],\"Top\":[{\"id\":\"Pm\",\"label\":\"P\",\"type\":\"output\"},{\"id\":\"Qm\",\"label\":\"Q\",\"type\":\"output\"}]}"
  RLC (Three-Phase) : ee_lib/Passive/RLC Assemblies/RLC (Three-Phase)  port_option=ee.enum.threePhasePort.composite  component_structure=ee.enum.rlc.structure.SeriesRL  R=filterResistance %5e-5 Ohm  L=filterInductance%0.00012 H  C=1e-6 F  R_parasitic=0 Ohm  G_parasitic=0 1/Ohm  IL_specify=on  IL_priority=None  IL=[0, 0, 0] A  IL_nominal_specify=off  IL_nominal_value=1  IL_nominal_unit=A  VC_specify=off  VC_priority=High  VC=[0, 0, 0] V  VC_nominal_specify=off  VC_nominal_value=1  VC_nominal_unit=V
      settings: InternalSimscapePortConfiguration="{\"Bottom\":[],\"Left\":[{\"id\":\"N1\",\"label\":\"~1\",\"type\":\"foundation.electrical.three_phase\"}],\"Right\":[{\"id\":\"N2\",\"label\":\"~2\",\"type\":\"foundation.electrical.three_phase\"}],\"Top\":[]}"
  In : PMIOPort  Side=Left
  ~ : PMIOPort  Port=2  Side=Right
  VIBus : Outport
  Out Bus Element : Outport  Port=2  PortName=Meas  Element=voltage
  Out Bus Element1 : Outport  Port=2  PortName=Meas  Element=current
  Out Bus Element2 : Outport  Port=2  PortName=Meas  Element=activePower
  Out Bus Element3 : Outport  Port=2  PortName=Meas  Element=reactivePower
  BusElementOut : Outport  Port=2  PortName=Meas  Element=SOC
  BusElementOut1 : Outport  Port=2  PortName=Meas  Element=Vdc
  BusElementOut2 : Outport  Port=2  PortName=Meas  Element=IBatt
  BusElementOut3 : Outport  Port=2  PortName=Meas  Element=Idc
  BusElementOut4 : Outport  Port=2  PortName=Meas  Element=ILoad
  BusElementOut5 : Outport  Port=2  PortName=Meas  Element=IDCDC
  BusElementOut6 : Outport  Port=2  PortName=Meas  Element=UPSBrK
  BusElementOut7 : Outport  Port=2  PortName=Meas  Element=rmsVoltage
  wires:
  BusElementIn/1 -> BusElementOut/1
  Gain1/1 -> Delay2/1
  Gain/1 -> Delay1/1
  PS-Simulink Converter2/1 -> Out Bus Element/1, Low-Pass Filter (Discrete or Continuous)2/1
  PS-Simulink Converter6/1 -> Low-Pass Filter (Discrete or Continuous)1/1
  PS-Simulink Converter7/1 -> Low-Pass Filter (Discrete or Continuous)/1
  PS-Simulink Converter3/1 -> Out Bus Element1/1, Low-Pass Filter (Discrete or Continuous)3/1
  Low-Pass Filter (Discrete or Continuous)/1 -> Gain1/1
  Low-Pass Filter (Discrete or Continuous)1/1 -> Gain/1
  PLL & Measurements/1(VIbus) -> Delay/1
  Delay/1 -> VIBus/1
  BusElementIn2/1 -> Gain3/1
  Delay1/1 -> Out Bus Element2/1
  Delay2/1 -> Out Bus Element3/1
  BusElementIn1/1 -> BusElementOut2/1
  Gain3/1 -> BusElementOut1/1
  BusElementIn3/1 -> BusElementOut3/1
  BusElementIn4/1 -> BusElementOut4/1
  Low-Pass Filter (Discrete or Continuous)2/1 -> PLL & Measurements/1(V)
  Low-Pass Filter (Discrete or Continuous)3/1 -> PLL & Measurements/2(I)
  BusElementIn5/1 -> BusElementOut5/1
  BusElementIn6/1 -> BusElementOut6/1
  PS-Simulink Converter4/1 -> BusElementOut7/1
  connections:
  Current and Voltage Sensor (Three-Phase)/RConn3 -- Power Sensor (Three-Phase)1/LConn1
  PS-Simulink Converter2/LConn1 -- Current and Voltage Sensor (Three-Phase)/RConn1 -- PS RMS Estimator/LConn1
  Current and Voltage Sensor (Three-Phase)/RConn2 -- PS-Simulink Converter3/LConn1
  Power Sensor (Three-Phase)1/LConn2 -- PS-Simulink Converter6/LConn1
  Power Sensor (Three-Phase)1/LConn3 -- PS-Simulink Converter7/LConn1
  Current and Voltage Sensor (Three-Phase)/LConn1 -- RLC (Three-Phase)/RConn1
  Power Sensor (Three-Phase)1/RConn1 -- ~/RConn1
  In/RConn1 -- RLC (Three-Phase)/LConn1
  PS-Simulink Converter4/LConn1 -- PS RMS Estimator/RConn1

== system UPS_Harness/UPS/Inverter/Inverter Controller ==
  VI : Inport
  Power : Inport  Port=2
  Current Limiter : Subsystem
  Droop Control : Subsystem  VariantControl=droop
  VoltageCurrentControl : Subsystem
  mabc : Outport
  wires:
  VI/1 -> VoltageCurrentControl/1(measure), Current Limiter/1(VI)
  VoltageCurrentControl/1(mabc) -> mabc/1
  Droop Control/2(Vqref) -> Current Limiter/3(Vq)
  Droop Control/1(Vdref) -> Current Limiter/2(Vd)
  Droop Control/3(omega) -> VoltageCurrentControl/6(w)
  Droop Control/4(Theta) -> VoltageCurrentControl/7(Angle)
  Current Limiter/3(Idmax) -> VoltageCurrentControl/4(Idmax)
  Current Limiter/2(VqRef) -> VoltageCurrentControl/3(Vqref)
  Current Limiter/1(VdRef) -> VoltageCurrentControl/2(Vdref)
  Current Limiter/4(Iqmax) -> VoltageCurrentControl/5(Iqmax)
  Power/1 -> Droop Control/1(Power)

== system UPS_Harness/UPS/Rectifier/Circuit Breaker ==
  BRK : Inport
  Data Type Conversion : DataTypeConversion  OutDataTypeStr=double  SaturateOnIntegerOverflow=off  RndMeth=Floor
  Open Resistance : Gain  Gain=5e7
  Phase Splitter : ee_lib/Connectors & References/Phase Splitter
  Phase Splitter1 : ee_lib/Connectors & References/Phase Splitter
  Simulink-PS Converter : nesl_utility/Simulink-PS Converter  PhysicalDomain=network_engine_domain  SubClassName=ps_input  LeftPortType=input  RightPortType=output  PseudoPeriodic=off  Frequencies=[]  NoiseDistribution=none  NoiseParameters=[]  Unit=1  AffineConversion=off  FilteringAndDerivatives=provide  SimscapeFilterOrder=1  InputFilterTimeConstant=0.001  UdotUserProvided=0
  Variable Resistor : fl_lib/Electrical/Electrical Elements/Variable Resistor  Rmin=1e-3 Ohm  thermalEnable=false  thermal_mass=1 J/K  i_specify=on  i_priority=None  i=0 A  i_nominal_specify=off  i_nominal_value=1  i_nominal_unit=A  v_specify=off  v_priority=None  v=0 V  v_nominal_specify=off  v_nominal_value=1  v_nominal_unit=V  T_specify=off  T_priority=None  T=300 K  T_nominal_specify=off  T_nominal_value=1  T_nominal_unit=K
  Variable Resistor1 : fl_lib/Electrical/Electrical Elements/Variable Resistor  Rmin=1e-3 Ohm  thermalEnable=false  thermal_mass=1 J/K  i_specify=on  i_priority=None  i=0 A  i_nominal_specify=off  i_nominal_value=1  i_nominal_unit=A  v_specify=off  v_priority=None  v=0 V  v_nominal_specify=off  v_nominal_value=1  v_nominal_unit=V  T_specify=off  T_priority=None  T=300 K  T_nominal_specify=off  T_nominal_value=1  T_nominal_unit=K
  Variable Resistor2 : fl_lib/Electrical/Electrical Elements/Variable Resistor  Rmin=1e-3 Ohm  thermalEnable=false  thermal_mass=1 J/K  i_specify=on  i_priority=None  i=0 A  i_nominal_specify=off  i_nominal_value=1  i_nominal_unit=A  v_specify=off  v_priority=None  v=0 V  v_nominal_specify=off  v_nominal_value=1  v_nominal_unit=V  T_specify=off  T_priority=None  T=300 K  T_nominal_specify=off  T_nominal_value=1  T_nominal_unit=K
  ABC2 : PMIOPort  Side=Left
  ~ : PMIOPort  Port=2  Side=Right
  wires:
  Data Type Conversion/1 -> Open Resistance/1
  BRK/1 -> Data Type Conversion/1
  Open Resistance/1 -> Simulink-PS Converter/1
  connections:
  Phase Splitter1/RConn2 -- Variable Resistor1/RConn1
  Variable Resistor1/LConn2 -- Phase Splitter/RConn2
  Phase Splitter1/RConn3 -- Variable Resistor2/RConn1
  Phase Splitter/RConn1 -- Variable Resistor/LConn2
  Variable Resistor2/LConn2 -- Phase Splitter/RConn3
  Phase Splitter1/RConn1 -- Variable Resistor/RConn1
  Phase Splitter1/LConn1 -- ~/RConn1
  Variable Resistor/LConn1 -- Simulink-PS Converter/RConn1 -- Variable Resistor2/LConn1 -- Variable Resistor1/LConn1
  Phase Splitter/LConn1 -- ABC2/RConn1
